simulink subsystem "LowLevelController"  (R2022b)
settings: Solver=VariableStepAuto  StartTime=0.0  StopTime=10.0  RelTol=1e-3
undefined symbols (not defined in the file): ProjectExample
settings Model: Creator=Ilya_Andriyanov  LastModifiedBy=user

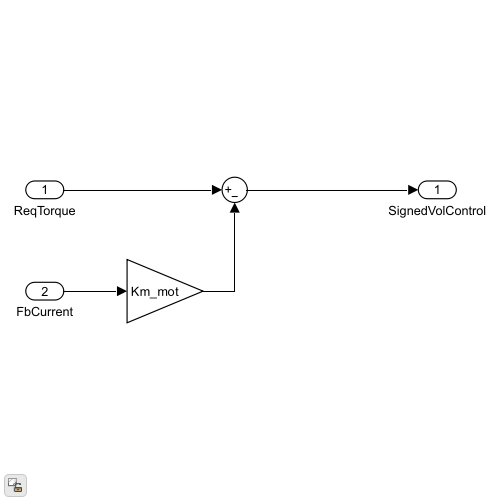
[thumbnail: Simulink's stored preview of the top-level diagram]
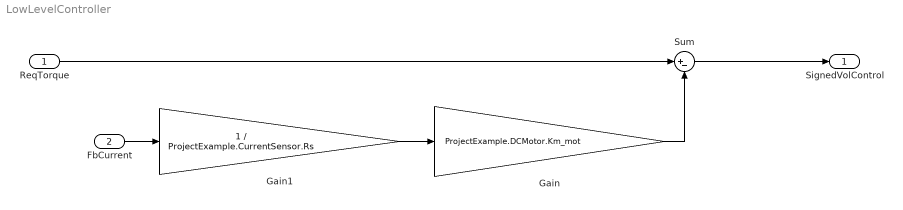
== system LowLevelController ==
  ReqTorque : Inport
  FbCurrent : Inport  Port=2
  Gain : Gain  Gain=ProjectExample.DCMotor.Km_mot
  Gain1 : Gain  Gain=1 / ProjectExample.CurrentSensor.Rs
  Sum : Sum  Inputs=|+-
  SignedVolControl : Outport
  wires:
  ReqTorque/1 -> Sum/1
  Sum/1 -> SignedVolControl/1
  FbCurrent/1 -> Gain1/1
  Gain/1 -> Sum/2
  Gain1/1 -> Gain/1
